simulink model "PPC_P2_fixed"  (R2019b)
settings: Solver=ode45  StartTime=0.0  StopTime=50.0  MaxStep=1.0  RelTol=1e-3
undefined symbols (not defined in the file or in its folder): sigbuilder_block
libraries: slctrlblks x1, simulink x1
settings Model: Creator=Kevin  LastModifiedBy=Kevin

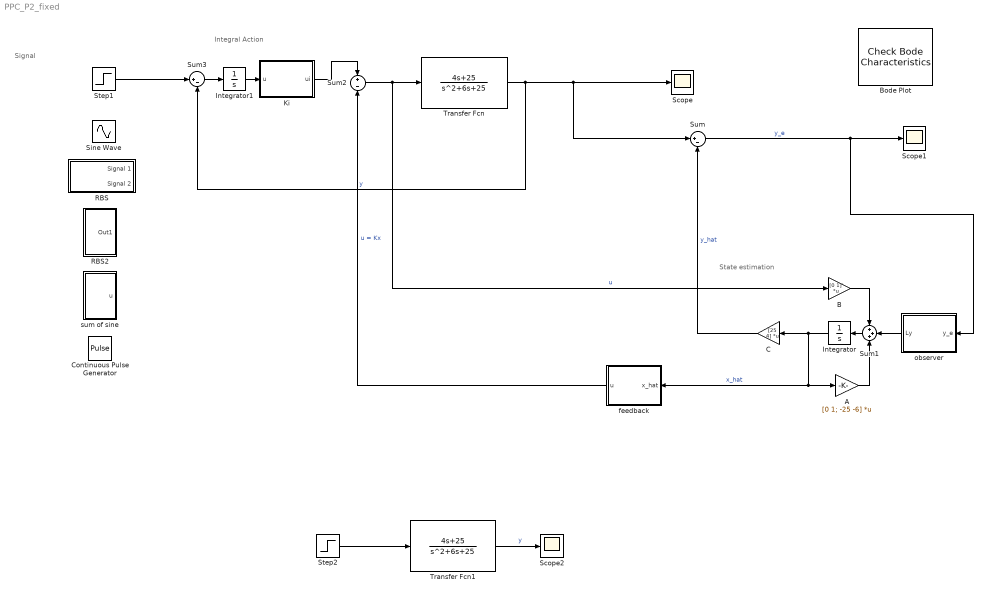
== system PPC_P2_fixed ==
  note: Integral Action
  note: Signal
  note: State estimation
  A : Gain  Gain=[0 1; -25 -6]  Multiplication=Matrix(K*u)
  B : Gain  Gain=[0 1]'  Multiplication=Matrix(K*u)
  Bode Plot : slctrlblks/Model Verification/Check Bode  Characteristics  InstantiateOnLoad=on  SaveOperatingPoints=off  LinearizationIOs={'/Sum2', 1, 'in', 'off', '';'/Transfer Fcn', 1, 'out', 'on', ''}  LinearizeAt=SnapshotTimes  SnapshotTimes=[0]  TriggerType=rising  SampleTime=auto  RateConversionMethod=zoh  PreWarpFreq=10  UseExactDelayModel=off  UseFullBlockNameLabels=off  UseBusSignalLabels=off  enabled=on  stopWhenAssertionFail=off  export=off  ViewDlgPos=[1921 -319 1920 967.333333333333]  OpenViewOnLoad=off  LaunchViewOnOpen=off  FrequencyUnits=rad/s  MagnitudeUnits=dB  PhaseUnits=deg  TimeUnits=seconds  EnableUpperBound=off  UpperBoundFrequencies=[]  UpperBoundMagnitudes=[]  EnableLowerBound=off  LowerBoundFrequencies=[]  LowerBoundMagnitudes=[]
      settings: SourceProductName=Simulink Control Design
  C : Gain  Gain=[25 4]  Multiplication=Matrix(K*u)
  Continuous Pulse Generator : DiscretePulseGenerator  PulseType=Time based  Period=1  PulseWidth=50
  Integrator : Integrator
  Integrator1 : Integrator
  Ki : MATLAB Function  TreatAsAtomicUnit=on
  "RBS " : Subsystem  Tag=STV Subsys  LoadFcn=sigbuilder_block('load');  StartFcn=sigbuilder_block('start');  StopFcn=sigbuilder_block('stop');  ClipboardFcn=sigbuilder_block('clipboard');  mask(Sigbuilder block){tuvar=[0:10]}
      mask help: Simulink:masks:SigbuilderBlock_MD
      mask init:
      | if ~strcmp(get_param(bdroot(gcbh),'SimulationStatus'),'stopped') tuvar = sigbuilder_block('maskInit'); end
      settings: CopyFcn=sigbuilder_block('copy');  DeleteFcn=sigbuilder_block('delete');  ModelCloseFcn=sigbuilder_block('modelClose');  PreSaveFcn=sigbuilder_block('preSave');  PauseFcn=sigbuilder_block('pause');  ContinueFcn=sigbuilder_block('continue');  NameChangeFcn=sigbuilder_block('namechange');  OpenFcn=sigbuilder_block('open',[215 62.5 550.5 362.5 ]);  CloseFcn=sigbuilder_block('close');
      mask Display: plot(0, 0, 100, 100,[2, 2, 32, 32, 2], [68, 8, 8, 68, 68],[32, 2], [38, 38], [32, 19, 2],[53, 60, 44], [32, 17, 17, 2],[16, 16, 31, 31]);txt = getActiveGroup(gcbh);text(2, 100, txt,'verticalAlignment', 'top');
  RBS2 : Subsystem
  Scope : Scope
  Scope1 : Scope
  Scope2 : Scope
  Sine Wave : Sin  Frequency=0.1  SampleTime=0
  Step1 : Step  SampleTime=0
  Step2 : Step  SampleTime=0
  Sum : Sum  Inputs=|+-
  Sum1 : Sum  Inputs=+++
  Sum2 : Sum  Inputs=+-
  Sum3 : Sum  Inputs=|+-
  Transfer Fcn : TransferFcn  Numerator=[4 25]  Denominator=[1 ,6 ,25]
  Transfer Fcn1 : TransferFcn  Numerator=[4 25]  Denominator=[1 ,6 ,25]
  feedback : MATLAB Function  TreatAsAtomicUnit=on
  "observer " : MATLAB Function  TreatAsAtomicUnit=on
  sum of sine : Subsystem
  wires:
  Transfer Fcn/1 -> Sum/1, Scope/1, Sum3/2  "y"
  Step1/1 -> Sum3/1
  Integrator1/1 -> Ki/1(u)
  Sum3/1 -> Integrator1/1
  Ki/1(ui) -> Sum2/1
  B/1 -> Sum1/1
  A/1 -> Sum1/3
  "observer "/1(Ly) -> Sum1/2
  Sum2/1 -> B/1, Transfer Fcn/1  "u"
  Integrator/1 -> C/1, feedback/1(x_hat), A/1  "x_hat"
  Sum/1 -> "observer "/1(y_e), Scope1/1  "y_e"
  C/1 -> Sum/2  "y_hat"
  Sum1/1 -> Integrator/1
  feedback/1(u) -> Sum2/2  "u = Kx"
  Step2/1 -> Transfer Fcn1/1
  Transfer Fcn1/1 -> Scope2/1  "y"

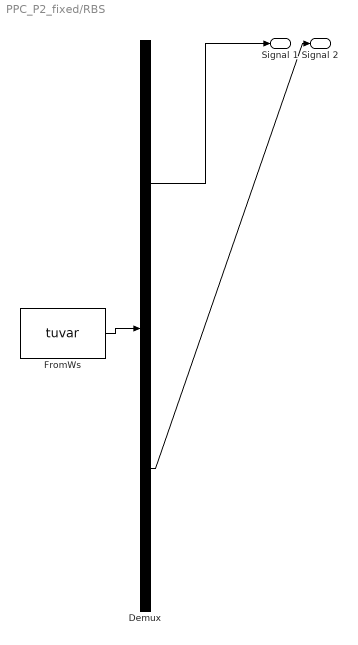
== system PPC_P2_fixed/RBS  ==
  Demux : Demux  Tag=STV Demux  Outputs=2
  FromWs : FromWorkspace  Tag=STV FromWs  VariableName=tuvar  SampleTime=0
      SigBuilderData=|
      | common.afterFinalStr = 'Extrapolate'
      | common.sampleTime = 0
      | dataSet.timeRange = [0 10]
      | dataSet.name = 'Group 1'
      | sbobj.Groups.Name = 'Group 1'
      | sbobj.Groups.Signals(1).Name = 'Signal 1'
      | sbobj.Groups.Signals(1).XData = [0 4 4 6 6 10]
      | sbobj.Groups.Signals(1).YData = [0 0 1 1 0 0]
      | sbobj.Groups.Signals(2).Name = 'Signal 2'
      | sbobj.Groups.Signals(2).XData = [0 0.2 0.2 0.3 0.3 0.5 0.5 0.7 0.7 1 1 1.1 1.1 1.3 1.3 1.4 1.4 1.5 1.5 1.7 1.7 2.1 2.1 2.2 2.2 2.7 2.7 2.8 2.8 2.9 2.9 3 3 3.1 3.1 3.5 3.5 3.7 3.7 3.8 3.8 3.9 3.9 4.2 4.2 4.4 4.4 4.7 4.7 5 5 5.1 5.1 5.3 5.3 5.6 5.6 5.7 5.7 5.8 5.8 5.9 5.9 6 6 6.1 6.1 6.2 6.2 6.7 6.7 7 7 7.1 7.1 7.2 7.2 7.3 7.3 7.4 7.4 7.5 7.5 7.8 7.8 7.9 7.9 8.1 8.1 8.5 8.5 8.6 8.6 8.8 8.8 8.9 8.9 9 9 9.2 9.2 9.5 9.5 9.6 9.6 9.7 9.7 10]
      | sbobj.Groups.Signals(2).YData = [1 1 0 0 1 1 0 0 1 1 0 0 1 1 0 0 1 1 0 0 1 1 0 0 1 1 0 0 1 1 0 0 1 1 0 0 1 1 0 0 1 1 0 0 1 1 0 0 1 1 0 0 1 1 0 0 1 1 0 0 1 1 0 0 1 1 0 0 1 1 0 0 1 1 0 0 1 1 0 0 1 1 0 0 1 1 0 0 1 1 0 0 1 1 0 0 1 1 0 0 1 1 0 0 1 1 0 0]
  Signal 1 : Outport  Tag=STV Outport
  Signal 2 : Outport  Tag=STV Outport  Port=2
  wires:
  Demux/1 -> Signal 1/1
  FromWs/1 -> Demux/1
  Demux/2 -> Signal 2/1

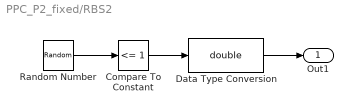
== system PPC_P2_fixed/RBS2 ==
  Compare To Constant : simulink/Logic and Bit Operations/Compare To Constant  relop=<=  const=1  OutDataTypeStr=boolean
  Data Type Conversion : DataTypeConversion  OutDataTypeStr=double
  Random Number : RandomNumber  Mean=1  SampleTime=10
  Out1 : Outport
  wires:
  Random Number/1 -> Compare To Constant/1
  Compare To Constant/1 -> Data Type Conversion/1
  Data Type Conversion/1 -> Out1/1

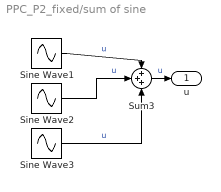
== system PPC_P2_fixed/sum of sine ==
  Sine Wave1 : Sin  Frequency=0.1  Phase=0.1  SampleTime=0
  Sine Wave2 : Sin  SampleTime=0
  Sine Wave3 : Sin  Frequency=2  SampleTime=0
  Sum3 : Sum  Inputs=+++
  u : Outport
  wires:
  Sine Wave3/1 -> Sum3/3  "u"
  Sine Wave1/1 -> Sum3/1  "u"
  Sum3/1 -> u/1  "u"
  Sine Wave2/1 -> Sum3/2  "u"

== matlab function PPC_P2_fixed/observer  ==
  data: y_e input; Ly output
function Ly  = fcn(y_e)
coder.extrinsic("ss","place","matsplit",'ctrb');
Ly = [0 0];
A = [0 1; -25 -6];
B = [0 1]';
C = [25 4]; 

%observer design
a0 = 25;
a1 = 6;
P = ctrb(A,B);
Pccf1 = [a1 1; 1 0];
p1 = -300; p2 = -300; 
alpha = [-(p1+p2) p1*p2];
L = [alpha(2)-a0 alpha(1)-a1]*inv(P*Pccf1);
Ly = L*y_e;

== matlab function PPC_P2_fixed/Ki ==
  data: u input; ui output
function ui = fcn(u)
 coder.extrinsic("ss","place","matsplit",'ctrb');
% [b2, b1, b0, a1, a0] = matsplit(theta);
ui = 0;
A = [0 1; -25 -6];
B = [0 1]';
C = [25 4]; 

o = [0 0]';
A1 = [A o;C 0];
B1 = [B;0];
p = [-30+4i -30-4i -10]; %let third pole be less affective
K1 = place(A1,B1,p);
Ki = [K1(3)];
ui = Ki*u;

== matlab function PPC_P2_fixed/feedback ==
  data: x_hat input; u output
function u = fcn(x_hat)
 coder.extrinsic("ss","place","matsplit",'ctrb');
% [b2, b1, b0, a1, a0] = matsplit(theta);
%[0 4 25 6 25]
% A = [0 1; -theta(5) -theta(4)];
% B = [0 1]';
% C = [theta(3) theta(2)];

K = [0 0];
u = 0;
A = [0 1; -25 -6];
B = [0 1]';
C = [25 4]; 

%servomechanism
o = [0 0]';
A1 = [A o;C 0];
B1 = [B;0];
%p = [-30+0.01i -30-0.01i -0.15]; %let third pole be less affective
p = [-30+4i -30-4i -10];
K1 = place(A1,B1,p);
K = [K1(1) K1(2)];
u = K*x_hat;
